simulink library "findTargetPathParameter"  (R2020a)
settings: Solver=VariableStepAuto  StartTime=0.0  StopTime=10.0  RelTol=1e-3
settings Model: Creator=Ayaz  LastModifiedBy=Ayaz

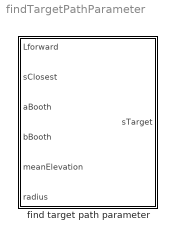
== system findTargetPathParameter ==
  find target path parameter : Subsystem

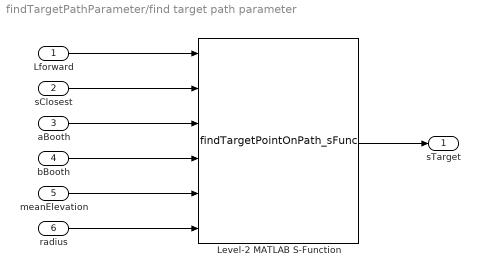
== system findTargetPathParameter/find target path parameter ==
  Lforward : Inport
  sClosest : Inport  Port=2
  aBooth : Inport  Port=3
  bBooth : Inport  Port=4
  meanElevation : Inport  Port=5
  radius : Inport  Port=6
  Level-2 MATLAB S-Function : M-S-Function  FunctionName=findTargetPointOnPath_sFunc
  sTarget : Outport
  wires:
  Level-2 MATLAB S-Function/1 -> sTarget/1
  aBooth/1 -> Level-2 MATLAB S-Function/3
  radius/1 -> Level-2 MATLAB S-Function/6
  sClosest/1 -> Level-2 MATLAB S-Function/2
  meanElevation/1 -> Level-2 MATLAB S-Function/5
  bBooth/1 -> Level-2 MATLAB S-Function/4
  Lforward/1 -> Level-2 MATLAB S-Function/1
